simulink model "Road_Simulink"  (R2018b)
settings: Solver=VariableStepAuto  StartTime=0.0  StopTime=19.99  RelTol=1e-3
values from neighbouring files (symbols this model uses):
  road_index = 1*ones(length(z_Smooth_LH),1)    [Road_Generator_Fullcar.m]    (also in Road_Generator_Fullcar_final.m = road_index(1:end-10); Road_Generator_Fullcar_symmetric.m = [3 * ones(length(z_Bump),1); 3 * ones(length(z_Bump),1); 3 *; Road_Generator_Quarter.m = [1 * ones(length(z_Smooth_LH),1); 2*ones(length(z_Rough_LH),; Road_Generator_Quarter_tester.m = [2 * ones(length(z_Smooth_LH),1); 1*ones(length(z_Rough_LH),)
  ROAD_x = x_Smooth    [Road_Generator_Fullcar.m]    (also in Road_Generator_Fullcar_final.m = ROAD_x(1:end-1); Road_Generator_Fullcar_symmetric.m = [x_Bump; Road_Generator_Quarter.m = [x_Rough; Road_Generator_Quarter_tester.m = [x_Smooth)
  ROAD_z_LH = z_Smooth_LH    [Road_Generator_Fullcar.m]    (also in Road_Generator_Fullcar_final.m = ROAD_z_LH(1:end-1); Road_Generator_Fullcar_symmetric.m = [z_Bump; z_Bump; z_Bump; z_Bump; z_Bump;]; Road_Generator_Quarter.m = [z_Rough_LH; z_Smooth_LH; z_Bump]; Road_Generator_Quarter_tester.m = [z_Smooth_LH; z_Rough_LH])
settings Model: Creator=6708742  LastModifiedBy=larban
settings SFSimCC: SimUseLocalCustomCode=off
settings RTWCC: RTWUseLocalCustomCode=off

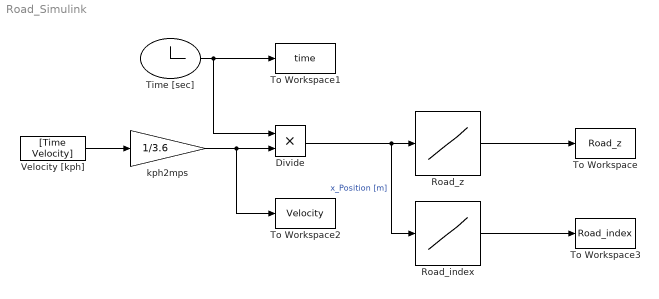
== system Road_Simulink ==
  Divide : Product  Inputs=**
  Road_index : Lookup_n-D  NumberOfTableDimensions=1  BreakpointsForDimension1=ROAD_x  Table=road_index  InternalRulePriority=Speed  RndMeth=Simplest  InputSameDT=on
  Road_z : Lookup_n-D  NumberOfTableDimensions=1  BreakpointsForDimension1=ROAD_x  Table=ROAD_z_LH  InternalRulePriority=Speed  RndMeth=Simplest  InputSameDT=on
  Time [sec] : Clock
      settings: Decimation=20
  To Workspace : ToWorkspace  VariableName=Road_z  SampleTime=0.01
  To Workspace1 : ToWorkspace  VariableName=time  SampleTime=0.01
  To Workspace2 : ToWorkspace  VariableName=Velocity  SampleTime=0.01
  To Workspace3 : ToWorkspace  VariableName=Road_index  SampleTime=0.01
  Velocity [kph] : FromWorkspace  VariableName=[Time Velocity]  SampleTime=0.001
  kph2mps : Gain  Gain=1/3.6
  wires:
  Velocity [kph]/1 -> kph2mps/1
  Divide/1 -> Road_index/1, Road_z/1  "x_Position [m]"
  Time [sec]/1 -> To Workspace1/1, Divide/1
  kph2mps/1 -> To Workspace2/1, Divide/2
  Road_z/1 -> To Workspace/1
  Road_index/1 -> To Workspace3/1
